simulink model "Cartesian_Control_second"  (R2021a)
settings: Solver=VariableStepAuto  StartTime=0.0  StopTime=20  RelTol=1e-3
libraries: robotmaniplib x4, robotcorelib x2
settings Model: Creator=ASUS  LastModifiedBy=ASUS

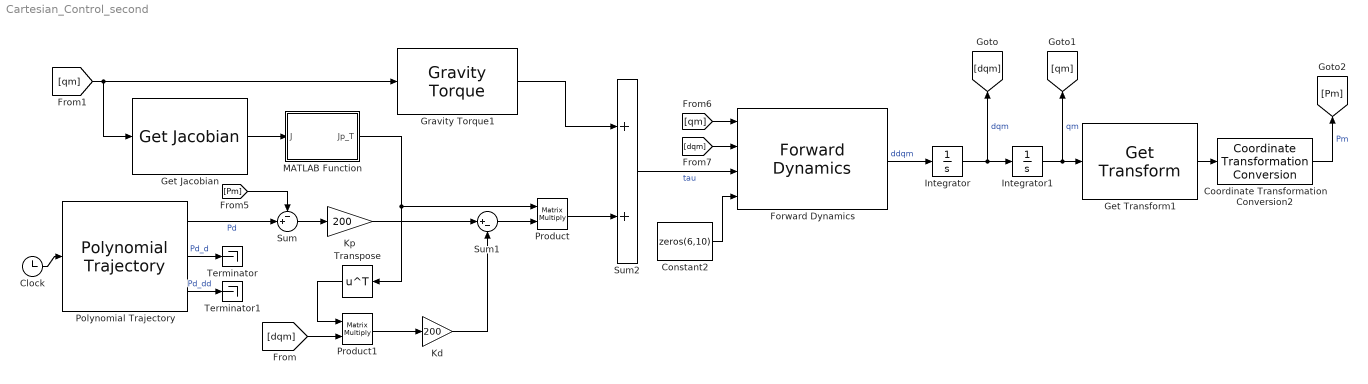
== system Cartesian_Control_second ==
  Clock : Clock
  Constant2 : Constant  Value=zeros(6,10)
  Coordinate Transformation Conversion2 : robotcorelib/Coordinate Transformation Conversion  InputRepresentation=Homogeneous Transformation  InputEulerSequence=ZYX  ShowTrVecInputPort=on  OutputRepresentation=Translation Vector  OutputEulerSequence=ZYX  ShowTrVecOutputPort=on  SimulateUsing=Code generation
      settings: SourceProductBaseCode=NV,RO,RR,UV
  Forward Dynamics : robotmaniplib/Forward Dynamics  RigidBodyTree=robot  SimulateUsing=Code generation
  Get Jacobian : robotmaniplib/Get Jacobian  RigidBodyTree=robot  EndEffector=tool0  SimulateUsing=Code generation
      settings: SourceProductBaseCode=RO
  Get Transform1 : robotmaniplib/Get Transform  RigidBodyTree=robot  SourceBody=tool0  TargetBody=world  SimulateUsing=Code generation
  Gravity Torque1 : robotmaniplib/Gravity Torque  RigidBodyTree=robot  SimulateUsing=Code generation
  Integrator : Integrator
  Integrator1 : Integrator
  Kd : Gain  Gain=200
  Kp : Gain  Gain=200
  MATLAB Function : MATLAB Function  TreatAsAtomicUnit=on
  Polynomial Trajectory : robotcorelib/Polynomial Trajectory  WaypointSource=Internal  Waypoints=[ 0.1 0.1; 0.2 0.2; 0.3 0.3]  TimePoints=[ 0, 0.01 ]  TimeInterval=[ 1, 4 ]  Method=Cubic Polynomial  ParameterSource=Internal  VelocityBoundaryCondition=zeros( 3, 2 )  AccelerationBoundaryCondition=zeros( 2, 5 )  SimulateUsing=Interpreted execution
  Product : Product  Multiplication=Matrix(*)
  Product1 : Product  Multiplication=Matrix(*)
  Sum : Sum  Inputs=-+|
  Sum1 : Sum  Inputs=|+-
  Sum2 : Sum
  Terminator : Terminator
  Terminator1 : Terminator
  Transpose : Math  Operator=transpose  SaturateOnIntegerOverflow=on
  wires:
  Clock/1 -> Polynomial Trajectory/1
  Forward Dynamics/1 -> Integrator/1  "ddqm"
  Integrator/1 -> [dqm], Integrator1/1  "dqm"
  Sum/1 -> Kp/1
  Constant2/1 -> Forward Dynamics/4
  Sum2/1 -> Forward Dynamics/3  "tau"
  Integrator1/1 -> Get Transform1/1, [qm]  "qm"
  Polynomial Trajectory/1 -> Sum/2  "Pd"
  [Pm] -> Sum/1
  [qm] -> Forward Dynamics/1
  [dqm] -> Forward Dynamics/2
  Gravity Torque1/1 -> Sum2/1
  Get Transform1/1 -> Coordinate Transformation Conversion2/1
  Coordinate Transformation Conversion2/1 -> [Pm]  "Pm"
  Get Jacobian/1 -> MATLAB Function/1(J)
  Polynomial Trajectory/3 -> Terminator1/1  "Pd_dd"
  Polynomial Trajectory/2 -> Terminator/1  "Pd_d"
  Product1/1 -> Kd/1
  [qm] -> Gravity Torque1/1, Get Jacobian/1
  Product/1 -> Sum2/2
  MATLAB Function/1(Jp_T) -> Transpose/1, Product/1
  [dqm] -> Product1/2
  Kd/1 -> Sum1/2
  Kp/1 -> Sum1/1
  Sum1/1 -> Product/2
  Transpose/1 -> Product1/1

== matlab function Cartesian_Control_second/MATLAB Function ==
  data: J input; Jp_T output
function Jp_T = fcn(J)

Jp_T = J(4:6,:)';

end
